simulink model "order1_MRAC"  (R2015b)
settings: Solver=ode45  StartTime=0.0  StopTime=20  RelTol=1e-3
settings Model: Creator=Administrator  LastModifiedBy=Sayan Basu Roy
settings DataIOCC: SaveFormat=Array
settings DebuggingCC: SolverPrmCheckMsg=warning
settings HardwareCC: ProdBitPerPointer=32  ProdLargestAtomicFloat=None  ProdIntDivRoundTo=Undefined  ProdEndianess=Unspecified  ProdWordSize=32  ProdHWDeviceType=32-bit Generic
settings GRTTargetCC: GeneratePreprocessorConditionals=Disable all
settings ConfigComp: CovModelRefEnable=Off  CovSFcnEnable=off

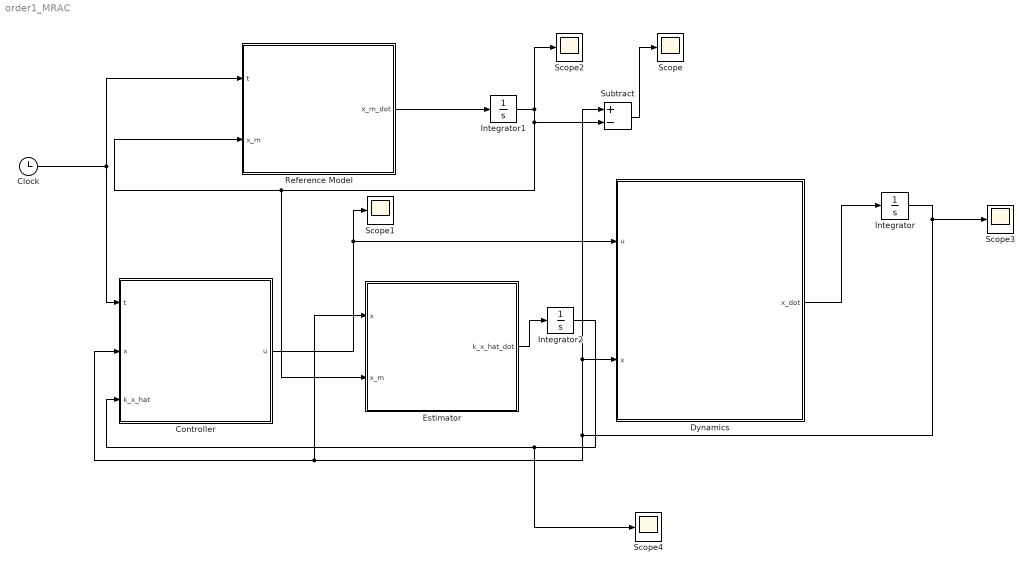
== system order1_MRAC ==
  Clock : Clock
      settings: Decimation=50
  Controller : MATLAB Function  TreatAsAtomicUnit=on
  Dynamics : MATLAB Function  TreatAsAtomicUnit=on
  Estimator : MATLAB Function  TreatAsAtomicUnit=on
  Integrator : Integrator  InitialCondition=10
  Integrator1 : Integrator  InitialCondition=10
  Integrator2 : Integrator
  Reference Model : MATLAB Function  TreatAsAtomicUnit=on
  Scope{,1..4} (5 alike) : Scope
  Subtract : Sum  Inputs=+-
  wires:
  Dynamics/1(x_dot) -> Integrator/1
  Integrator/1 -> Scope3/1, Subtract/1, Dynamics/2(x), Estimator/1(x), Controller/2(x)
  Clock/1 -> Controller/1(t), Reference Model/1(t)
  Controller/1(u) -> Scope1/1, Dynamics/1(u)
  Reference Model/1(x_m_dot) -> Integrator1/1
  Integrator1/1 -> Scope2/1, Estimator/2(x_m), Reference Model/2(x_m), Subtract/2
  Estimator/1(k_x_hat_dot) -> Integrator2/1
  Integrator2/1 -> Scope4/1, Controller/3(k_x_hat)
  Subtract/1 -> Scope/1

== matlab function order1_MRAC/Controller ==
  data: u output; t input; x input; k_x_hat input
function u  = controller(t,x,k_x_hat)

%r=10;
%r=exp(-t);
r=0;
u=k_x_hat*x+r;

end

== matlab function order1_MRAC/Dynamics ==
  data: u input; x input; x_dot output
function x_dot   = dynamics(u,x)
%#codegen
a=-1;
b=2;
x_dot=a*x+b*u;
end

== matlab function order1_MRAC/Estimator ==
  data: k_x_hat_dot output; x input; x_m input
function k_x_hat_dot  = estimator(x,x_m)

e=x-x_m;
b=2;
gamma=0.1;



k_x_hat_dot=-gamma*e*b*x;

== matlab function order1_MRAC/Reference Model ==
  data: x_m_dot output; t input; x_m input
function x_m_dot  = reference(t,x_m)
a_m=-2;
b_m=2;
%r=exp(-t);
r=0;

x_m_dot=a_m*x_m+b_m*r;
